simulink model "graph_import"  (R2023a)
settings: Solver=VariableStepAuto  StartTime=0.0  StopTime=10  RelTol=1e-3
undefined symbols (not defined in the file): AIE, ML, S, vsvh1760, xcve2802
libraries: aieBasic x1, simulink x1, vmcUtilities x1, dspsrcs4 x1, aieUtilities x1
settings Model: Creator=abehbood  LastModifiedBy=robg
settings SolverCC: AlgebraicLoopSolver=TrustRegion
settings DebuggingCC: UnconnectedInputMsg=warning  UnconnectedOutputMsg=warning  UnconnectedLineMsg=warning
settings ModelReferenceCC: EnableRefExpFcnMdlSchedulingChecks=on
settings RTWCC: DLArmComputeVersion=19.05

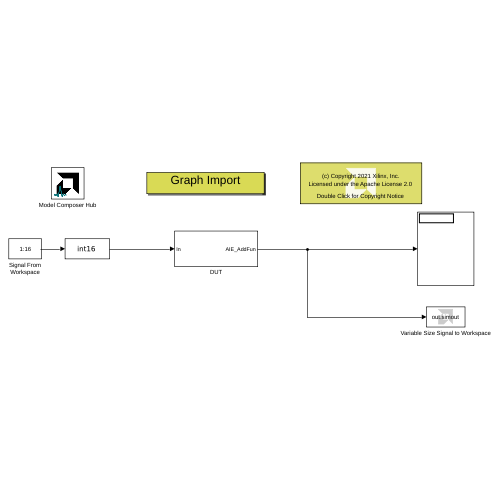
[thumbnail: Simulink's stored preview of the top-level diagram]
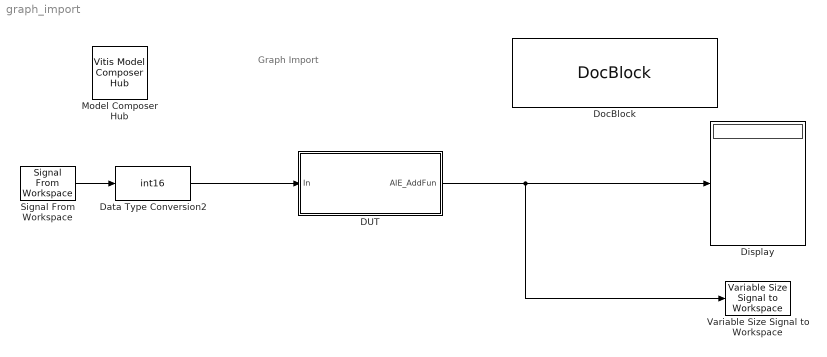
== system graph_import ==
  note: Graph Import
  DUT : Subsystem
  Data Type Conversion2 : DataTypeConversion  OutDataTypeStr=int16  SaturateOnIntegerOverflow=off  RndMeth=Floor
  Display : Display
  DocBlock : simulink/Model-Wide Utilities/DocBlock  DocumentType=Text  mask(DocBlock){}
      mask Display:
      | xmcDrawBlockIcon();
      | disp(['{\fontsize{10pt}(c) Copyright 2021' ' Xilinx, Inc.}\newline \newline '],'texmode','on');
      | disp('{\fontsize{10pt}Licensed under the Apache License 2.0}','texmode','on');
      | disp('\newline \newline \newline{\fontsize{10pt}Double Click for Copyright Notice}','texmode','on');
  Model Composer Hub : vmcUtilities/Vitis Model Composer Hub  Tag=genX  CodeGeneration=off  SubsystemName=DUT  StartColumn=1  NumberOfColumns=1  TargetDirectory=./code  exportDesign=off  analyzeDesign=off  validateDesignOnHw=off  ExportType=AI Engines  IpVendor=xilinx.com  IpLibrary=hls  IpVersion=1.0  IpHWLanguage=Verilog  AieCompilerOptions={}  AieSimulatorOptions={}  CreateTestbench=on  TestbenchStackSize=10  RunRtlSim=off  RunCSim=off  RunAieSim=on  AieSimTimeout=50000  RunAieSimProfiling=off  LaunchVitisAnalyzer=off  PlotOutput=off  RunX86Sim=off  X86SimTimeout=10  GenHwImage=off  GenLibadfXo=off  GenHwValidationCode=off  PlatformType=Not Specified  HwSystemType=Baremetal  HwValidationTarget=hw  ProjDevice=xcve2802-vsvh1760-2LP-e-S  ProjDevicePart=xcve2802-vsvh1760-2LP-e-S  AIEType=AIE-ML  SamplePeriod=-1  ClockFrequency=200  DataPathParallelism=1  xilinxfamily=versalaiedge  part=xcve2802  speed=-2LP-e-S  package=vsvh1760  directory=./netlist  testbench=off  incr_netlist=off  synthesis_tool=Vivado  clock_wrapper=Clock Enables  dbl_ovrd=According to Block Masks  dcm_input_clock_period=10  sysclk_period=10  simulink_period=1  eval_field=0  IPInfoJsonString="{\"AIESubsystem\":{\"SubsystemName\":\"DUT\",\"TargetDirectory\":\"./code\",\"SubsystemDir\":\"./code/ip/DUT\"}}"  LogFileName=/proj/xsjhdstaff4/abehbood/vmc_examples/gitent2/Examples/AIENGINE/Importing_AIE_blocks/AIE_Graph/code/model_composer.log  NThreads=4
  Signal From Workspace : dspsrcs4/Signal From Workspace  X=1:16  Ts=1  nsamps=16  OutputAfterFinalValue=Setting to zero  ignoreOrWarnInputAndFrameLengths=off  OutputFrames=off
  Variable Size Signal to Workspace : aieUtilities/Variable Size Signal to Workspace  VariableNameMask=simout
  wires:
  DUT/1(AIE_AddFun) -> Display/1, Variable Size Signal to Workspace/1
  Data Type Conversion2/1 -> DUT/1(In)
  Signal From Workspace/1 -> Data Type Conversion2/1

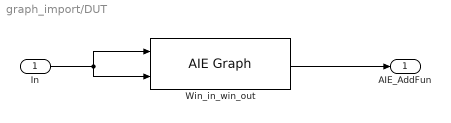
== system graph_import/DUT ==
  In : Inport
  Win_in_win_out : aieBasic/AIE Graph  PortAttributesTable={ 'Input', 'In1', 'buffer', 'int16', '16', 'sync', ''; 'Input', 'In2', 'buffer', 'int16', '16', 'sync', ''; 'Output', 'Out1', 'buffer', 'int16', '16', 'sync', '' }  PortAttributesEnablement={'off', 'on', 'off', 'off', 'off', 'off', 'off';'off', 'on', 'off', 'off', 'off', 'off', 'off';'off', 'on', 'off', 'off', 'off', 'off', 'off'}  SampleTime=-1  ClassDeclTypeOptions=C[1 1]@t20@class Win_in_win_out  ClassDecl=class Win_in_win_out  ClassTemplateParams={}  ClassTemplateParamsEnables={}  ClassCtorDeclTypeOptions=C[1 1]@t7@<empty>  ClassCtorDecl=<empty>  ClassCtorParams={}  GraphAllAttrs=|  PortArgDecls={'in buffer int16 in1'; 'in buffer int16 in2'; 'out buffer int16 out1'}  PortGraphPortNames={'In1'; 'In2'; 'Out1'}  HierGraphPortNames={'In1'; 'In2'; 'Out1'}  PortTypes={'buffer'; 'buffer'; 'buffer'}  PortDataTypes={'int16'; 'int16'; 'int16'}  PortSizes={1.600000000000000000e+01; 1.600000000000000000e+01; 1.600000000000000000e+01}  PortSynchronicities={'sync'; 'sync'; 'sync'}  PortSignalSizes={0.000000000000000000e+00; 0.000000000000000000e+00; 0.000000000000000000e+00}  SimLibPath=''  ClassIndex=1  ClassCtorIndex=0  ClassTabVisible=off  FunctionTabVisible=on  DelayDrawLabels=off  GraphFileSelect=Header file (*.h)  GraphHeaderFile=win_in_win_out.h  GraphClassName=Win_in_win_out  GraphName=Win_in_win_out  GraphHeaderFiles={'./win_in_win_out.h'}  GraphSourceFile=./model_composer_work/xmc_aie_lib/a79ee908/mygraph.cpp  GraphSearchPaths={'./src/kernels/', './src/kernels'}  GraphPreProcOptions={}  blockJsonConstraints=[]
      | s[12;12;9;9;19;14;21;23;21;23;24;21;15;17;12;24;26;26;26;27;28;9;21;23;23;23;24;25;14;19;19;29]@FunctionNameDeclFileNamePortNamesPortTypesPortSerializedTypesPortDirectionsPortWindowSizeEnablesPortWindowMarginEnablesPortBufferSizeEnablesPortBufferMarginEnablesPortSynchronicityEnablesPortSignalSizeEnablesPortBufferSizesPortBufferMarginsFunctionDeclFunctionTemplateSpecKindFunctionTemplateParamNamesFunctionTemplateParamKindsFunctionTemplateParamTypesFunctionTemplateParamValuesFunctionTemplateParamEnablesClassDeclClassTemplateSpecKindClassTemplateParamNamesClassTemplateParamKindsClassTemplateParamTypesClassTemplateParamValuesClassTemplateParamEnablesClassCtorDeclsClassCtorParamNamesClassCtorParamTypesClassCtorParamSerializedTypes[1 1]@C[32 1]@nt22@../../win_in_win_out.hC[3 1]@t3@In1t3@In2t4@Out1C[3 1]@t31@adf::port< adf::direction::in >t31@adf::port< adf::direction::in >t32@adf::port< adf::direction::out >C[3 1]@t39@{Tadf::port{1{t{Sadf::direction::in}}}}t39@{Tadf::port{1{t{Sadf::direction::in}}}}t40@{Tadf::port{1{t{Sadf::direction::out}}}}C[3 1]@t5@inputt5@inputt5@inputC[3 1]@l0@l0@l0@C[3 1]@l0@l0@l0@C[3 1]@l0@l0@l0@C[3 1]@l0@l0@l0@C[3 1]@l1@l1@l1@C[3 1]@l0@l0@l0@C[3 1]@nnnC[3 1]@nnnt135@void Win_in_win_out::
      | (adf::port< adf::direction::in > In1, adf::port< adf::direction::in > In2, adf::port< adf::direction::out > Out1)ne[0 1]@e[0 1]@e[0 1]@e[0 1]@e[0 1]@t21@class Win_in_win_out;t4@nonee[0 1]@e[0 1]@e[0 1]@e[0 1]@e[0 1]@e[0 1]@e[0 1]@e[0 1]@e[0 1]@
  AIE_AddFun : Outport
  wires:
  In/1 -> Win_in_win_out/2, Win_in_win_out/1
  Win_in_win_out/1 -> AIE_AddFun/1
